simulink model "Sursa_Nestabilizata"  (R2020a)
settings: Solver=VariableStepAuto  StartTime=0.0  StopTime=0.5  RelTol=1e-3
settings Model: Creator=Stefi  LastModifiedBy=Stefi

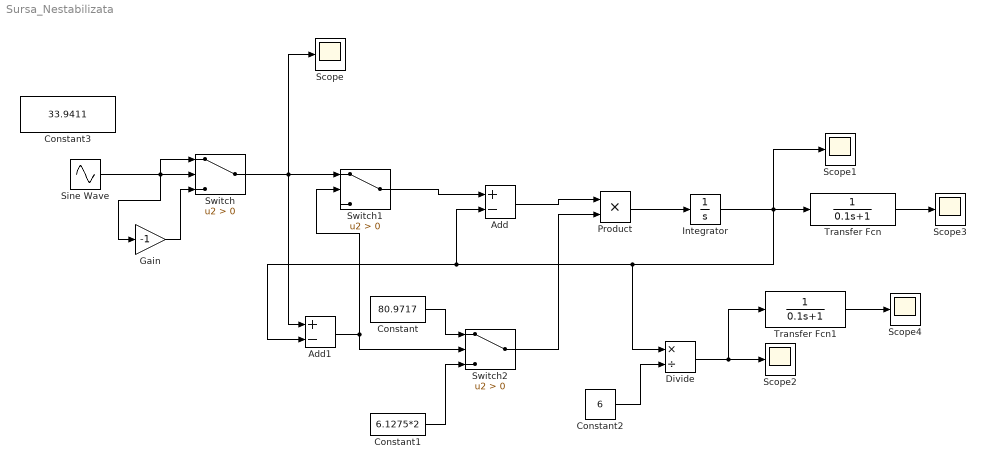
== system Sursa_Nestabilizata ==
  Add : Sum  Inputs=+-
  Add1 : Sum  Inputs=+-
  Constant : Constant  Value=80.9717
  Constant1 : Constant  Value=6.1275*2
  Constant2 : Constant  Value=6
  Constant3 : Constant  Value=33.9411
  Divide : Product  Inputs=*/
  Gain : Gain  Gain=-1
  Integrator : Integrator
  Product : Product
  Scope{,1..4} (5 alike) : Scope
      Scope settings: Tag=Scope
  Sine Wave : Sin  Amplitude=33.9411  Frequency=314  SampleTime=0
  Switch : Switch  Criteria=u2 > Threshold
  Switch1 : Switch  Criteria=u2 > Threshold
  Switch2 : Switch  Criteria=u2 > Threshold
  Transfer Fcn : TransferFcn  Denominator=[0.1 1]
  Transfer Fcn1 : TransferFcn  Denominator=[0.1 1]
  wires:
  Sine Wave/1 -> Gain/1, Switch/1, Switch/2
  Gain/1 -> Switch/3
  Switch/1 -> Add1/1, Scope/1, Switch1/1
  Switch1/1 -> Add/1
  Add/1 -> Product/1
  Product/1 -> Integrator/1
  Integrator/1 -> Divide/1, Add/2, Add1/2, Transfer Fcn/1, Scope1/1
  Add1/1 -> Switch2/2, Switch1/2
  Constant/1 -> Switch2/1
  Constant1/1 -> Switch2/3
  Switch2/1 -> Product/2
  Constant2/1 -> Divide/2
  Divide/1 -> Transfer Fcn1/1, Scope2/1
  Transfer Fcn/1 -> Scope3/1
  Transfer Fcn1/1 -> Scope4/1
